simulink model "ACC"  (R2020b)
settings: Solver=VariableStepAuto  StartTime=0.0  StopTime=500  RelTol=1e-3
values from neighbouring files (symbols this model uses):
  plant_den = [1 1/50.531]    [ACC_Script.m]
  plant_num = 9.2251*1e-4    (= 0.00092251)    [ACC_Script.m]    (also in Cruise_Control_design.m; Headway_Controller_Design.m = 0.00092212)
undefined symbols (not defined in the file or in its folder): sigbuilder_block
libraries: pid_lib x2
settings Model: Creator=ChOm1  LastModifiedBy=ChOm1

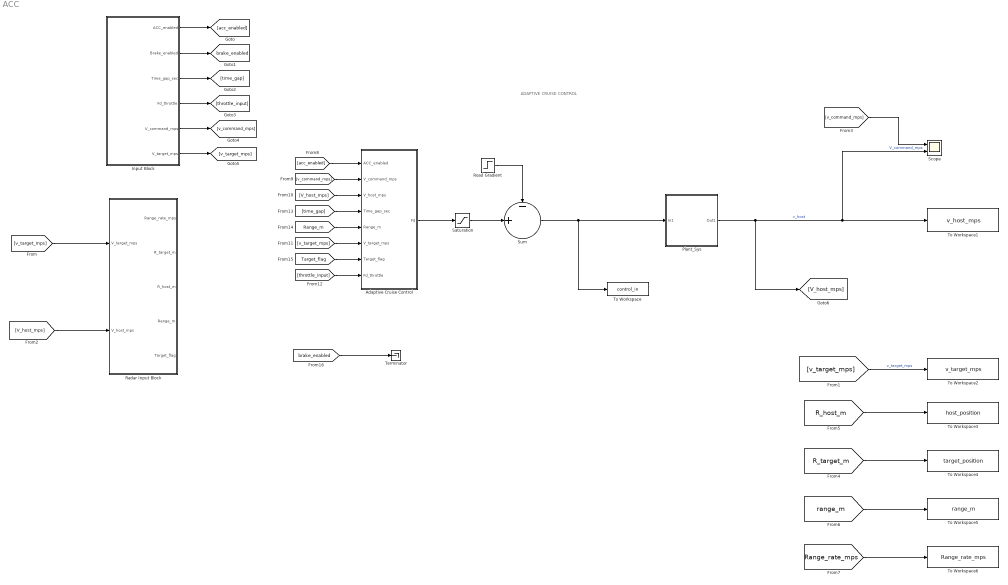
== system ACC ==
  note: ADAPTIVE CRUISE CONTROL
  Adaptive Cruise Control : Subsystem
  Input Block : Subsystem
  Plant_Sys : Subsystem
  Radar Input Block : Subsystem
  Road Gradient : Step  SampleTime=0
  Saturation : Saturate  UpperLimit=1000  LowerLimit=-1000
  Scope : Scope  NumInputPorts=2
  Sum : Sum  Inputs=-+|
  Terminator : Terminator
  To Workspace : ToWorkspace  VariableName=control_in  SaveFormat=Timeseries  SampleTime=-1
  To Workspace1 : ToWorkspace  VariableName=v_host_mps  SaveFormat=Timeseries  SampleTime=-1
  To Workspace2 : ToWorkspace  VariableName=v_target_mps  SaveFormat=Timeseries  SampleTime=-1
  To Workspace3 : ToWorkspace  VariableName=host_position  SaveFormat=Timeseries  SampleTime=-1
  To Workspace4 : ToWorkspace  VariableName=target_position  SaveFormat=Timeseries  SampleTime=-1
  To Workspace5 : ToWorkspace  VariableName=range_m  SaveFormat=Timeseries  SampleTime=-1
  To Workspace6 : ToWorkspace  VariableName=Range_rate_mps  SaveFormat=Timeseries  SampleTime=-1
  tag scope: brake_enabled=global
  wires:
  Input Block/1(ACC_enabled) -> [acc_enabled]
  Input Block/2(Brake_enabled) -> [brake_enabled]
  Input Block/3(Time_gap_sec) -> [time_gap]
  Input Block/4(Fd_throttle) -> [throttle_input]
  Input Block/5(V_command_mps) -> [v_command_mps]
  Input Block/6(V_target_mps) -> [v_target_mps]
  [v_target_mps] -> Radar Input Block/1(V_target_mps)
  Adaptive Cruise Control/1(Fd) -> Saturation/1
  Saturation/1 -> Sum/2
  Road Gradient/1 -> Sum/1
  Plant_Sys/1(Out1) -> [V_host_mps], Scope/2, To Workspace1/1  "v_host"
  [v_target_mps] -> To Workspace2/1  "v_target_mps"
  [v_command_mps] -> Scope/1  "V_command_mps"
  [R_target_m] -> To Workspace4/1
  [R_host_m] -> To Workspace3/1
  [range_m] -> To Workspace5/1
  [Range_rate_mps] -> To Workspace6/1
  [acc_enabled] -> Adaptive Cruise Control/1(ACC_enabled)
  [v_command_mps] -> Adaptive Cruise Control/2(V_command_mps)
  [V_host_mps] -> Adaptive Cruise Control/3(V_host_mps)
  [v_target_mps] -> Adaptive Cruise Control/6(V_target_mps)
  [throttle_input] -> Adaptive Cruise Control/8(Fd_throttle)
  [time_gap] -> Adaptive Cruise Control/4(Time_gap_sec)
  [Range_m] -> Adaptive Cruise Control/5(Range_m)
  [Target_flag] -> Adaptive Cruise Control/7(Target_flag)
  [brake_enabled] -> Terminator/1
  Sum/1 -> Plant_Sys/1(In1), To Workspace/1
  [V_host_mps] -> Radar Input Block/2(V_host_mps)

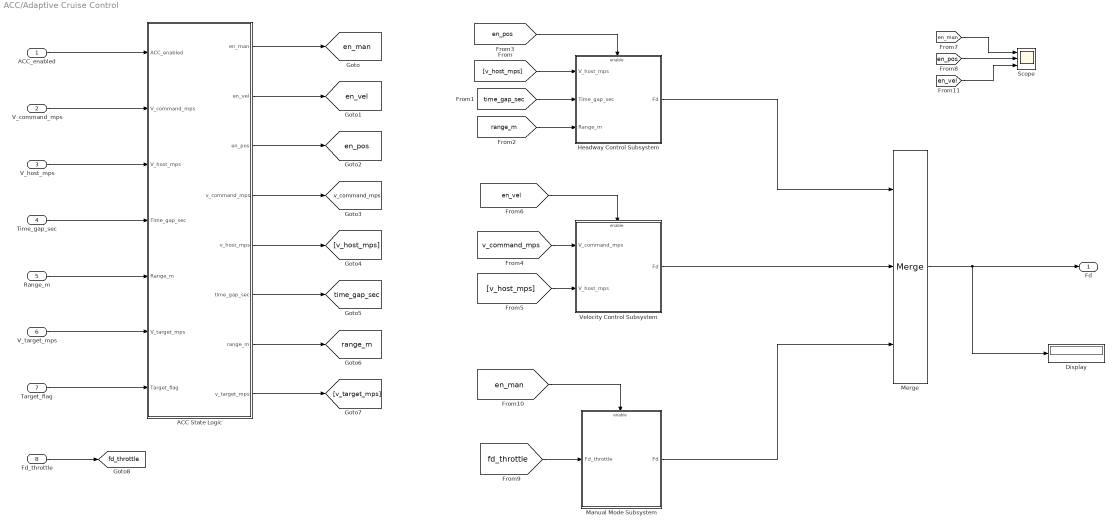
== system ACC/Adaptive Cruise Control ==
  ACC_enabled : Inport
  V_command_mps : Inport  Port=2
  V_host_mps : Inport  Port=3
  Time_gap_sec : Inport  Port=4
  Range_m : Inport  Port=5
  V_target_mps : Inport  Port=6
  Target_flag : Inport  Port=7
  Fd_throttle : Inport  Port=8
  ACC State Logic : Subsystem
  Display : Display
  Headway Control Subsystem : Subsystem
  Manual Mode Subsystem : Subsystem
  Merge : Merge  Inputs=3
  Scope : Scope  NumInputPorts=3
  Velocity Control Subsystem : Subsystem
  Fd : Outport
  tag scope: en_man=global, en_pos=global, en_vel=global, fd_throttle=global, range_m=global, time_gap_sec=global, v_command_mps=global
  wires:
  ACC_enabled/1 -> ACC State Logic/1(ACC_enabled)
  V_command_mps/1 -> ACC State Logic/2(V_command_mps)
  V_host_mps/1 -> ACC State Logic/3(V_host_mps)
  Time_gap_sec/1 -> ACC State Logic/4(Time_gap_sec)
  Range_m/1 -> ACC State Logic/5(Range_m)
  V_target_mps/1 -> ACC State Logic/6(V_target_mps)
  Target_flag/1 -> ACC State Logic/7(Target_flag)
  ACC State Logic/1(en_man) -> [en_man]
  ACC State Logic/2(en_vel) -> [en_vel]
  ACC State Logic/3(en_pos) -> [en_pos]
  ACC State Logic/4(v_command_mps) -> [v_command_mps]
  ACC State Logic/5(v_host_mps) -> [v_host_mps]
  ACC State Logic/6(time_gap_sec) -> [time_gap_sec]
  ACC State Logic/7(range_m) -> [range_m]
  ACC State Logic/8(v_target_mps) -> [v_target_mps]
  [v_host_mps] -> Headway Control Subsystem/1(V_host_mps)
  [time_gap_sec] -> Headway Control Subsystem/2(Time_gap_sec)
  [range_m] -> Headway Control Subsystem/3(Range_m)
  [en_pos] -> Headway Control Subsystem/Enable
  [v_command_mps] -> Velocity Control Subsystem/1(V_command_mps)
  [v_host_mps] -> Velocity Control Subsystem/2(V_host_mps)
  [en_vel] -> Velocity Control Subsystem/Enable
  Fd_throttle/1 -> [fd_throttle]
  [fd_throttle] -> Manual Mode Subsystem/1(Fd_throttle)
  [en_man] -> Manual Mode Subsystem/Enable
  Headway Control Subsystem/1(Fd) -> Merge/1
  Velocity Control Subsystem/1(Fd) -> Merge/2
  Manual Mode Subsystem/1(Fd) -> Merge/3
  Merge/1 -> Display/1, Fd/1
  [en_man] -> Scope/1
  [en_pos] -> Scope/2
  [en_vel] -> Scope/3

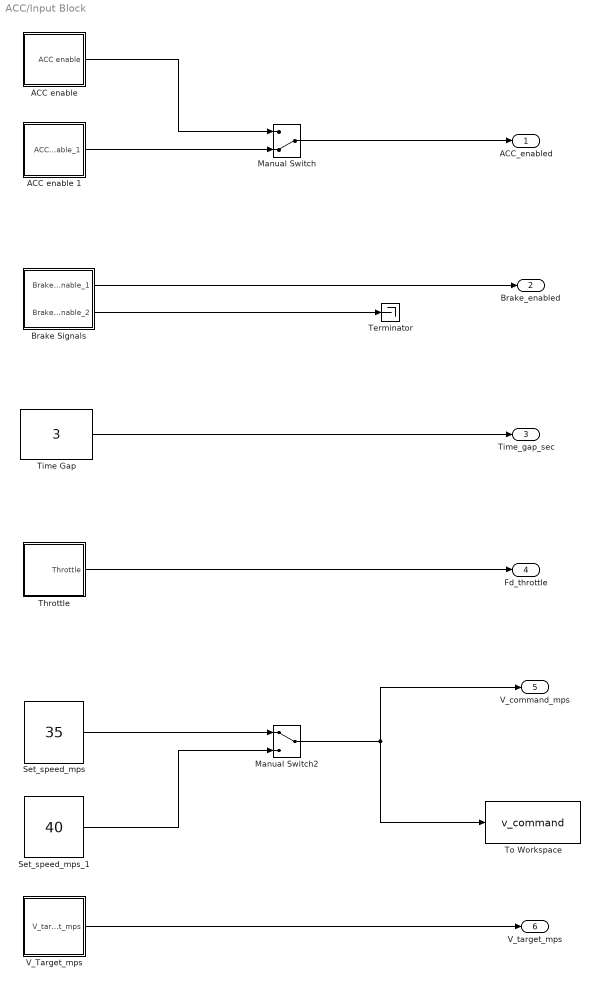
== system ACC/Input Block ==
  ACC enable : Subsystem  Tag=STV Subsys  LoadFcn=sigbuilder_block('load');  StartFcn=sigbuilder_block('start');  StopFcn=sigbuilder_block('stop');  ClipboardFcn=sigbuilder_block('clipboard');  mask(Sigbuilder block){tuvar=[0:10]}
      mask help: Simulink:masks:SigbuilderBlock_MD
      mask init:
      | if ~strcmp(get_param(bdroot(gcbh),'SimulationStatus'),'stopped') tuvar = sigbuilder_block('maskInit'); end
      settings: CopyFcn=sigbuilder_block('copy');  DeleteFcn=sigbuilder_block('delete');  ModelCloseFcn=sigbuilder_block('modelClose');  PreSaveFcn=sigbuilder_block('preSave');  PauseFcn=sigbuilder_block('pause');  ContinueFcn=sigbuilder_block('continue');  NameChangeFcn=sigbuilder_block('namechange');  OpenFcn=sigbuilder_block('open',[172.5 40 550.5 362.5 ]);  CloseFcn=sigbuilder_block('close');
      mask Display: plot(0, 0, 100, 100,[2, 2, 32, 32, 2], [68, 8, 8, 68, 68],[32, 2], [38, 38], [32, 19, 2],[53, 60, 44], [32, 17, 17, 2],[16, 16, 31, 31]);txt = getActiveGroup(gcbh);text(2, 100, txt,'verticalAlignment', 'top');
  ACC enable 1 : Subsystem  Tag=STV Subsys  LoadFcn=sigbuilder_block('load');  StartFcn=sigbuilder_block('start');  StopFcn=sigbuilder_block('stop');  ClipboardFcn=sigbuilder_block('clipboard');  mask(Sigbuilder block){tuvar=[0:10]}
      mask help: Simulink:masks:SigbuilderBlock_MD
      mask init:
      | if ~strcmp(get_param(bdroot(gcbh),'SimulationStatus'),'stopped') tuvar = sigbuilder_block('maskInit'); end
      settings: CopyFcn=sigbuilder_block('copy');  DeleteFcn=sigbuilder_block('delete');  ModelCloseFcn=sigbuilder_block('modelClose');  PreSaveFcn=sigbuilder_block('preSave');  PauseFcn=sigbuilder_block('pause');  ContinueFcn=sigbuilder_block('continue');  NameChangeFcn=sigbuilder_block('namechange');  OpenFcn=sigbuilder_block('open',[427 63 479.5 302.5 ]);  CloseFcn=sigbuilder_block('close');
      mask Display: plot(0, 0, 100, 100,[2, 2, 32, 32, 2], [68, 8, 8, 68, 68],[32, 2], [38, 38], [32, 19, 2],[53, 60, 44], [32, 17, 17, 2],[16, 16, 31, 31]);txt = getActiveGroup(gcbh);text(2, 100, txt,'verticalAlignment', 'top');
  Brake Signals : Subsystem  Tag=STV Subsys  LoadFcn=sigbuilder_block('load');  StartFcn=sigbuilder_block('start');  StopFcn=sigbuilder_block('stop');  ClipboardFcn=sigbuilder_block('clipboard');  mask(Sigbuilder block){tuvar=[0:10]}
      mask help: Simulink:masks:SigbuilderBlock_MD
      mask init:
      | if ~strcmp(get_param(bdroot(gcbh),'SimulationStatus'),'stopped') tuvar = sigbuilder_block('maskInit'); end
      settings: CopyFcn=sigbuilder_block('copy');  DeleteFcn=sigbuilder_block('delete');  ModelCloseFcn=sigbuilder_block('modelClose');  PreSaveFcn=sigbuilder_block('preSave');  PauseFcn=sigbuilder_block('pause');  ContinueFcn=sigbuilder_block('continue');  NameChangeFcn=sigbuilder_block('namechange');  OpenFcn=sigbuilder_block('open',[87.5 9 430.5 307 ]);  CloseFcn=sigbuilder_block('close');
      mask Display: plot(0, 0, 100, 100,[2, 2, 32, 32, 2], [68, 8, 8, 68, 68],[32, 2], [38, 38], [32, 19, 2],[53, 60, 44], [32, 17, 17, 2],[16, 16, 31, 31]);txt = getActiveGroup(gcbh);text(2, 100, txt,'verticalAlignment', 'top');
  Manual Switch : ManualSwitch  CurrentSetting=0
  Manual Switch2 : ManualSwitch
  Set_speed_mps : Constant  Value=35
  Set_speed_mps_1 : Constant  Value=40
  Terminator : Terminator
  Throttle : Subsystem  Tag=STV Subsys  LoadFcn=sigbuilder_block('load');  StartFcn=sigbuilder_block('start');  StopFcn=sigbuilder_block('stop');  ClipboardFcn=sigbuilder_block('clipboard');  mask(Sigbuilder block){tuvar=[0:10]}
      mask help: Simulink:masks:SigbuilderBlock_MD
      mask init:
      | if ~strcmp(get_param(bdroot(gcbh),'SimulationStatus'),'stopped') tuvar = sigbuilder_block('maskInit'); end
      settings: CopyFcn=sigbuilder_block('copy');  DeleteFcn=sigbuilder_block('delete');  ModelCloseFcn=sigbuilder_block('modelClose');  PreSaveFcn=sigbuilder_block('preSave');  PauseFcn=sigbuilder_block('pause');  ContinueFcn=sigbuilder_block('continue');  NameChangeFcn=sigbuilder_block('namechange');  OpenFcn=sigbuilder_block('open',[172.5 40 550.5 362.5 ]);  CloseFcn=sigbuilder_block('close');
      mask Display: plot(0, 0, 100, 100,[2, 2, 32, 32, 2], [68, 8, 8, 68, 68],[32, 2], [38, 38], [32, 19, 2],[53, 60, 44], [32, 17, 17, 2],[16, 16, 31, 31]);txt = getActiveGroup(gcbh);text(2, 100, txt,'verticalAlignment', 'top');
  Time Gap : Constant  Value=3
  To Workspace : ToWorkspace  VariableName=v_command  SaveFormat=Timeseries  SampleTime=-1
  V_Target_mps : Subsystem  Tag=STV Subsys  LoadFcn=sigbuilder_block('load');  StartFcn=sigbuilder_block('start');  StopFcn=sigbuilder_block('stop');  ClipboardFcn=sigbuilder_block('clipboard');  mask(Sigbuilder block){tuvar=[0:10]}
      mask help: Simulink:masks:SigbuilderBlock_MD
      mask init:
      | if ~strcmp(get_param(bdroot(gcbh),'SimulationStatus'),'stopped') tuvar = sigbuilder_block('maskInit'); end
      settings: CopyFcn=sigbuilder_block('copy');  DeleteFcn=sigbuilder_block('delete');  ModelCloseFcn=sigbuilder_block('modelClose');  PreSaveFcn=sigbuilder_block('preSave');  PauseFcn=sigbuilder_block('pause');  ContinueFcn=sigbuilder_block('continue');  NameChangeFcn=sigbuilder_block('namechange');  OpenFcn=sigbuilder_block('open',[5.5 30 949 418 ]);  CloseFcn=sigbuilder_block('close');
      mask Display: plot(0, 0, 100, 100,[2, 2, 32, 32, 2], [68, 8, 8, 68, 68],[32, 2], [38, 38], [32, 19, 2],[53, 60, 44], [32, 17, 17, 2],[16, 16, 31, 31]);txt = getActiveGroup(gcbh);text(2, 100, txt,'verticalAlignment', 'top');
  ACC_enabled : Outport
  Brake_enabled : Outport  Port=2
  Time_gap_sec : Outport  Port=3
  Fd_throttle : Outport  Port=4
  V_command_mps : Outport  Port=5
  V_target_mps : Outport  Port=6
  wires:
  Manual Switch/1 -> ACC_enabled/1
  Brake Signals/1(Brake_enable_1) -> Brake_enabled/1
  Brake Signals/2(Brake_enable_2) -> Terminator/1
  Time Gap/1 -> Time_gap_sec/1
  Throttle/1(Throttle) -> Fd_throttle/1
  V_Target_mps/1(V_target_mps) -> V_target_mps/1
  ACC enable/1(ACC enable) -> Manual Switch/1
  ACC enable 1/1(ACC_enable_1) -> Manual Switch/2
  Set_speed_mps/1 -> Manual Switch2/1
  Manual Switch2/1 -> To Workspace/1, V_command_mps/1
  Set_speed_mps_1/1 -> Manual Switch2/2

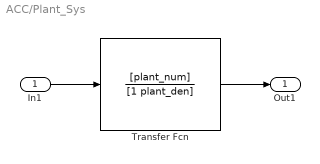
== system ACC/Plant_Sys ==
  In1 : Inport
  Transfer Fcn : TransferFcn  Numerator=[plant_num]  Denominator=[1 plant_den]
  Out1 : Outport
  wires:
  In1/1 -> Transfer Fcn/1
  Transfer Fcn/1 -> Out1/1

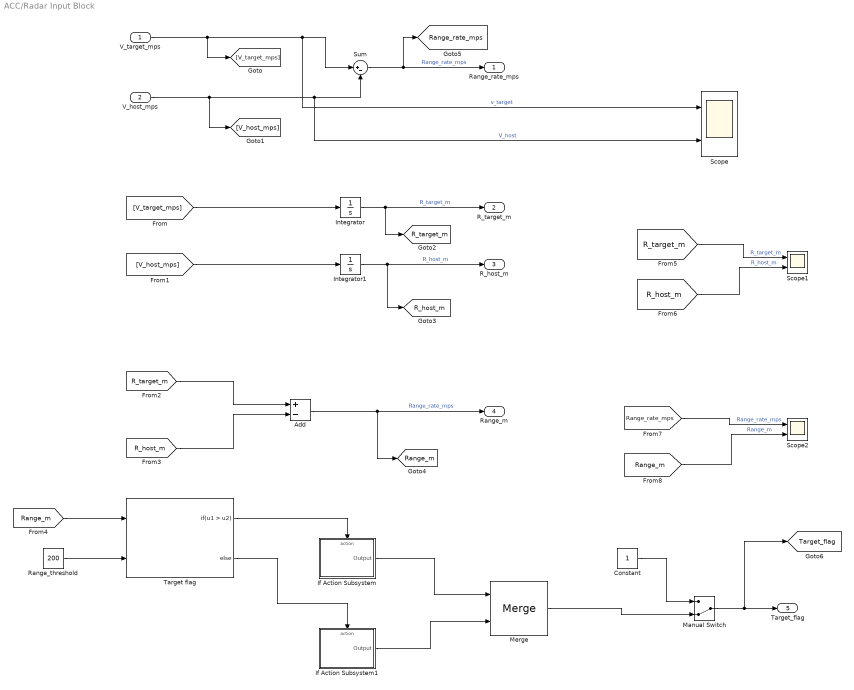
== system ACC/Radar Input Block ==
  V_target_mps : Inport
  V_host_mps : Inport  Port=2
  Add : Sum  Inputs=+-
  Constant : Constant
  If Action Subsystem : Subsystem  TreatAsAtomicUnit=on
  If Action Subsystem1 : Subsystem  TreatAsAtomicUnit=on
  Integrator : Integrator  InitialCondition=500
  Integrator1 : Integrator
  Manual Switch : ManualSwitch  CurrentSetting=0
  Merge : Merge
  Range_threshold : Constant  Value=200
  Scope : Scope  NumInputPorts=2
  Scope1 : Scope  NumInputPorts=2
  Scope2 : Scope  NumInputPorts=2
  Sum : Sum  Inputs=|+-
  "Target flag " : If  NumInputs=2  IfExpression=u1 > u2
  Range_rate_mps : Outport
  R_target_m : Outport  Port=2
  R_host_m : Outport  Port=3
  Range_m : Outport  Port=4
  Target_flag : Outport  Port=5
  tag scope: R_host_m=global, R_target_m=global, Range_m=global, Range_rate_mps=global, Target_flag=global
  wires:
  V_host_mps/1 -> [V_host_mps], Scope/2, Sum/2  "V_host"
  V_target_mps/1 -> Scope/1, Sum/1, [V_target_mps]  "v_target"
  Sum/1 -> [Range_rate_mps], Range_rate_mps/1  "Range_rate_mps"
  [V_target_mps] -> Integrator/1
  [V_host_mps] -> Integrator1/1
  Integrator1/1 -> [R_host_m], R_host_m/1  "R_host_m"
  Integrator/1 -> [R_target_m], R_target_m/1  "R_target_m"
  [R_target_m] -> Add/1
  [R_host_m] -> Add/2
  Add/1 -> [Range_m], Range_m/1  "Range_rate_mps"
  Range_threshold/1 -> "Target flag "/2
  [Range_m] -> "Target flag "/1
  "Target flag "/1 -> If Action Subsystem/Action
  "Target flag "/2 -> If Action Subsystem1/Action
  If Action Subsystem/1(Output) -> Merge/1
  If Action Subsystem1/1(Output) -> Merge/2
  Manual Switch/1 -> [Target_flag], Target_flag/1
  Constant/1 -> Manual Switch/1
  Merge/1 -> Manual Switch/2
  [R_target_m] -> Scope1/1  "R_target_m"
  [R_host_m] -> Scope1/2  "R_host_m"
  [Range_rate_mps] -> Scope2/1  "Range_rate_mps"
  [Range_m] -> Scope2/2  "Range_m"

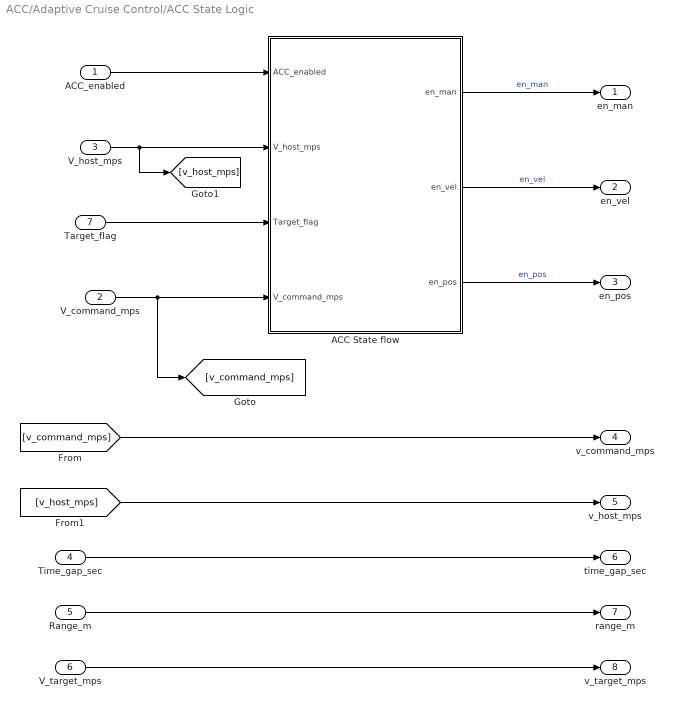
== system ACC/Adaptive Cruise Control/ACC State Logic ==
  ACC_enabled : Inport
  V_command_mps : Inport  Port=2
  V_host_mps : Inport  Port=3
  Time_gap_sec : Inport  Port=4
  Range_m : Inport  Port=5
  V_target_mps : Inport  Port=6
  Target_flag : Inport  Port=7
  ACC State flow : Stateflow chart  TreatAsAtomicUnit=on
  en_man : Outport
  en_vel : Outport  Port=2
  en_pos : Outport  Port=3
  v_command_mps : Outport  Port=4
  v_host_mps : Outport  Port=5
  time_gap_sec : Outport  Port=6
  range_m : Outport  Port=7
  v_target_mps : Outport  Port=8
  wires:
  ACC State flow/2(en_vel) -> en_vel/1  "en_vel"
  ACC State flow/3(en_pos) -> en_pos/1  "en_pos"
  [v_command_mps] -> v_command_mps/1
  [v_host_mps] -> v_host_mps/1
  Time_gap_sec/1 -> time_gap_sec/1
  Range_m/1 -> range_m/1
  V_target_mps/1 -> v_target_mps/1
  ACC State flow/1(en_man) -> en_man/1  "en_man"
  ACC_enabled/1 -> ACC State flow/1(ACC_enabled)
  Target_flag/1 -> ACC State flow/3(Target_flag)
  V_host_mps/1 -> [v_host_mps], ACC State flow/2(V_host_mps)
  V_command_mps/1 -> [v_command_mps], ACC State flow/4(V_command_mps)

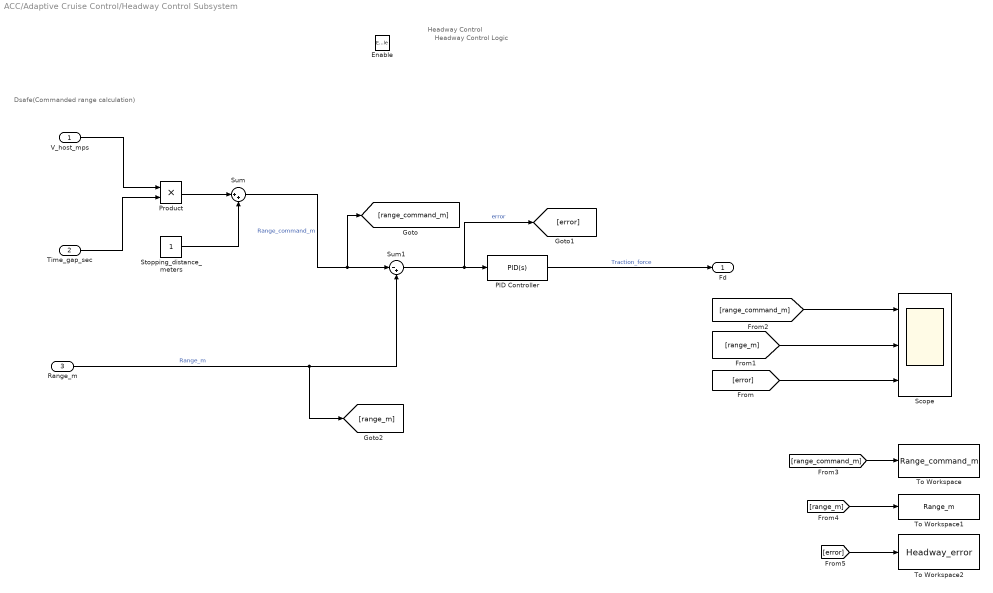
== system ACC/Adaptive Cruise Control/Headway Control Subsystem ==
  note: Headway Control Logic
  note: Headway Control
  note: Dsafe(Commanded range calculation)
  V_host_mps : Inport
  Time_gap_sec : Inport  Port=2
  Range_m : Inport  Port=3
  Enable : EnablePort
  PID Controller : pid_lib/PID Controller  Controller=PID  Form=Parallel  TimeDomain=Continuous-time  UseExternalTs=off  SampleTime=-1  IntegratorMethod=Forward Euler  FilterMethod=Forward Euler  ControllerParametersSource=internal  P=1.23373996546318  I=0.00611903694432425  D=34.7378082281947  UseFilter=on  N=75  TunerSelectOption=Transfer Function Based (PID Tuner App)  InitialConditionSource=internal  InitialConditionForIntegrator=0  InitialConditionForFilter=0  DifferentiatorICPrevScaledInput=0  ExternalReset=none  TrackingMode=off  Kt=1  LimitOutput=off  SatLimitsSource=internal  UpperSaturationLimit=inf  LowerSaturationLimit=-inf  LinearizeAsGain=on  AntiWindupMode=none  Kb=1  POutMin=[]  POutMax=[]  IOutMin=[]  IOutMax=[]  DOutMin=[]  DOutMax=[]  NOutMin=[]  NOutMax=[]  SumOutMin=[]  SumOutMax=[]  SaturationOutMin=[]  SaturationOutMax=[]  PParamMin=[]  PParamMax=[]  IParamMin=[]  IParamMax=[]  DParamMin=[]  DParamMax=[]  NParamMin=[]  NParamMax=[]  KbParamMin=[]  KbParamMax=[]  KtParamMin=[]  KtParamMax=[]  KbOutMin=[]  KbOutMax=[]  KtOutMin=[]  KtOutMax=[]  IntegratorOutMin=[]  IntegratorOutMax=[]  FilterOutMin=[]  FilterOutMax=[]  SumI1OutMin=[]  SumI1OutMax=[]  SumI2OutMin=[]  SumI2OutMax=[]  SumI3OutMin=[]  SumI3OutMax=[]  SumI4OutMin=[]  SumI4OutMax=[]  SumDOutMin=[]  SumDOutMax=[]  DifferentiatorOutMin=[]  DifferentiatorOutMax=[]  FilterDiffOutCoefMin=[]  FilterDiffOutCoefMax=[]  ReciprocalOutMin=[]  ReciprocalOutMax=[]  SumDenOutMin=[]  SumDenOutMax=[]  SumNumOutMin=[]  SumNumOutMax=[]  DivideOutMin=[]  DivideOutMax=[]  UdiffTsProdOutMin=[]  UdiffTsProdOutMax=[]  NTsProdOutMin=[]  NTsProdOutMax=[]  UintegralTsProdOutMin=[]  UintegralTsProdOutMax=[]  UngainTsProdOutMin=[]  UngainTsProdOutMax=[]  IntegratorContinuousStateAttributes=''  IntegratorStateMustResolveToSignalObject=off  IntegratorRTWStateStorageClass=Auto  FilterContinuousStateAttributes=''  FilterStateMustResolveToSignalObject=off  FilterRTWStateStorageClass=Auto  ParallelPVariant=InternalParameters  IdealPVariant=Disabled  IVariant=InternalParameters  DVariant=InternalParameters  IntegratorVariant=Continuous  SatVariant=Disabled  AWVariant=Passthrough  PCopyVariant=Disabled  TRVariant=Disabled  FdbkBlocksVariant=Forward  IdealPFdbkVariant=Disabled  SatFdbkVariant=Disabled  DerivativeFilterVariant=ContFilter  NVariant=InternalParameters  NCopyVariant=Disabled  FilterICVariant=InternalICsFilter  IntegratorICVariant=InternalICs  ExternalResetVariant=Disabled  TRSumVariant=Passthrough  SumFdbkVariant=Disabled  SumVariant=Sum_PID  TsampFilterVariant=InternalTs  TsampNgainVariant=Passthrough  TsampIntegralVariant=Passthrough  ExternalSaturationOutDataTypeStr=Inherit: Same as second input
  Product : Product
  Scope : Scope  NumInputPorts=3
  Stopping_distance_meters : Constant
  Sum : Sum  Inputs=|++
  Sum1 : Sum  Inputs=|-+
  To Workspace : ToWorkspace  VariableName=Range_command_m  SampleTime=-1
  To Workspace1 : ToWorkspace  VariableName=Range_m  SampleTime=-1
  To Workspace2 : ToWorkspace  VariableName=Headway_error  SaveFormat=Timeseries  SampleTime=-1
  Fd : Outport
  wires:
  [range_m] -> To Workspace1/1
  [error] -> Scope/3
  [error] -> To Workspace2/1
  [range_command_m] -> Scope/1
  [range_m] -> Scope/2
  [range_command_m] -> To Workspace/1
  PID Controller/1 -> Fd/1  "Traction_force"
  Sum/1 -> [range_command_m], Sum1/1  "Range_command_m"
  Stopping_distance_meters/1 -> Sum/2
  V_host_mps/1 -> Product/1
  Sum1/1 -> [error], PID Controller/1  "error"
  Time_gap_sec/1 -> Product/2
  Range_m/1 -> [range_m], Sum1/2  "Range_m"
  Product/1 -> Sum/1

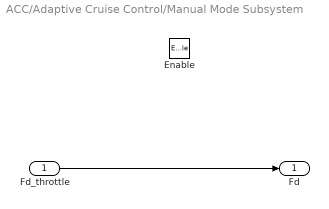
== system ACC/Adaptive Cruise Control/Manual Mode Subsystem ==
  Fd_throttle : Inport
  Enable : EnablePort
  Fd : Outport
  wires:
  Fd_throttle/1 -> Fd/1

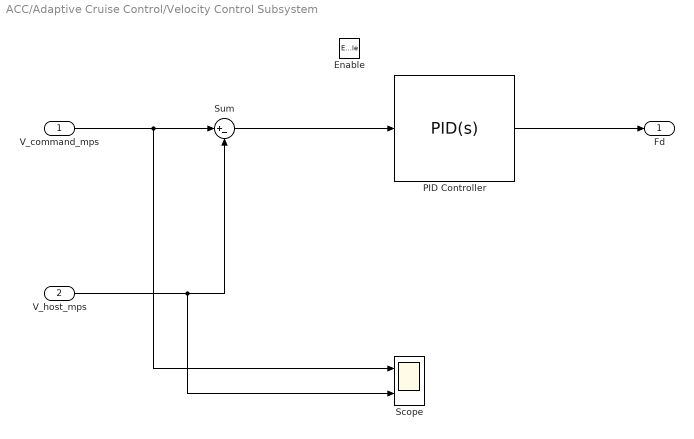
== system ACC/Adaptive Cruise Control/Velocity Control Subsystem ==
  V_command_mps : Inport
  V_host_mps : Inport  Port=2
  Enable : EnablePort
  PID Controller : pid_lib/PID Controller  Controller=PID  Form=Parallel  TimeDomain=Continuous-time  UseExternalTs=off  SampleTime=-1  IntegratorMethod=Forward Euler  FilterMethod=Forward Euler  ControllerParametersSource=internal  P=174.6119  I=10.1187  D=247.7833  UseFilter=on  N=100  TunerSelectOption=Transfer Function Based (PID Tuner App)  InitialConditionSource=internal  InitialConditionForIntegrator=0  InitialConditionForFilter=0  DifferentiatorICPrevScaledInput=0  ExternalReset=none  TrackingMode=off  Kt=1  LimitOutput=off  SatLimitsSource=internal  UpperSaturationLimit=inf  LowerSaturationLimit=-inf  LinearizeAsGain=on  AntiWindupMode=none  Kb=1  POutMin=[]  POutMax=[]  IOutMin=[]  IOutMax=[]  DOutMin=[]  DOutMax=[]  NOutMin=[]  NOutMax=[]  SumOutMin=[]  SumOutMax=[]  SaturationOutMin=[]  SaturationOutMax=[]  PParamMin=[]  PParamMax=[]  IParamMin=[]  IParamMax=[]  DParamMin=[]  DParamMax=[]  NParamMin=[]  NParamMax=[]  KbParamMin=[]  KbParamMax=[]  KtParamMin=[]  KtParamMax=[]  KbOutMin=[]  KbOutMax=[]  KtOutMin=[]  KtOutMax=[]  IntegratorOutMin=[]  IntegratorOutMax=[]  FilterOutMin=[]  FilterOutMax=[]  SumI1OutMin=[]  SumI1OutMax=[]  SumI2OutMin=[]  SumI2OutMax=[]  SumI3OutMin=[]  SumI3OutMax=[]  SumI4OutMin=[]  SumI4OutMax=[]  SumDOutMin=[]  SumDOutMax=[]  DifferentiatorOutMin=[]  DifferentiatorOutMax=[]  FilterDiffOutCoefMin=[]  FilterDiffOutCoefMax=[]  ReciprocalOutMin=[]  ReciprocalOutMax=[]  SumDenOutMin=[]  SumDenOutMax=[]  SumNumOutMin=[]  SumNumOutMax=[]  DivideOutMin=[]  DivideOutMax=[]  UdiffTsProdOutMin=[]  UdiffTsProdOutMax=[]  NTsProdOutMin=[]  NTsProdOutMax=[]  UintegralTsProdOutMin=[]  UintegralTsProdOutMax=[]  UngainTsProdOutMin=[]  UngainTsProdOutMax=[]  IntegratorContinuousStateAttributes=''  IntegratorStateMustResolveToSignalObject=off  IntegratorRTWStateStorageClass=Auto  FilterContinuousStateAttributes=''  FilterStateMustResolveToSignalObject=off  FilterRTWStateStorageClass=Auto  ParallelPVariant=InternalParameters  IdealPVariant=Disabled  IVariant=InternalParameters  DVariant=InternalParameters  IntegratorVariant=Continuous  SatVariant=Disabled  AWVariant=Passthrough  PCopyVariant=Disabled  TRVariant=Disabled  FdbkBlocksVariant=Forward  IdealPFdbkVariant=Disabled  SatFdbkVariant=Disabled  DerivativeFilterVariant=ContFilter  NVariant=InternalParameters  NCopyVariant=Disabled  FilterICVariant=InternalICsFilter  IntegratorICVariant=InternalICs  ExternalResetVariant=Disabled  TRSumVariant=Passthrough  SumFdbkVariant=Disabled  SumVariant=Sum_PID  TsampFilterVariant=InternalTs  TsampNgainVariant=Passthrough  TsampIntegralVariant=Passthrough  ExternalSaturationOutDataTypeStr=Inherit: Same as second input
  Scope : Scope  NumInputPorts=2
  Sum : Sum  Inputs=|+-
  Fd : Outport
  wires:
  V_host_mps/1 -> Scope/2, Sum/2
  V_command_mps/1 -> Scope/1, Sum/1
  Sum/1 -> PID Controller/1
  PID Controller/1 -> Fd/1

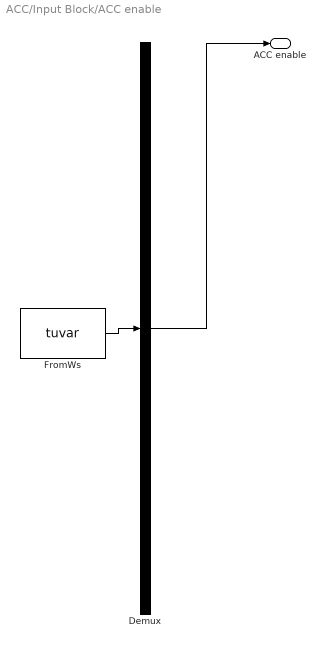
== system ACC/Input Block/ACC enable ==
  Demux : Demux  Tag=STV Demux  Outputs=1
      settings: DisplayOption=none
  FromWs : FromWorkspace  Tag=STV FromWs  VariableName=tuvar
      SigBuilderData=|
      | common.afterFinalStr = 'Extrapolate'
      | common.sampleTime = 0
      | dataSet.timeRange = [0 500]
      | dataSet.name = 'Group 1'
      | sbobj.Groups.Name = 'Group 1'
      | sbobj.Groups.Signals.Name = 'ACC enable'
      | sbobj.Groups.Signals.XData = [0 500]
      | sbobj.Groups.Signals.YData = [0.99 0.99]
      | sbobj.Groups.TimeRange = [0 500]
  ACC enable : Outport  Tag=STV Outport
  wires:
  FromWs/1 -> Demux/1
  Demux/1 -> ACC enable/1

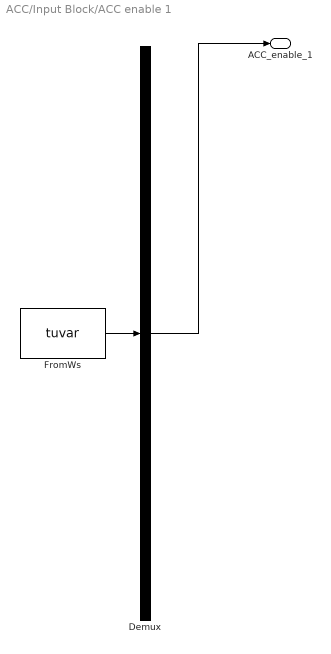
== system ACC/Input Block/ACC enable 1 ==
  Demux : Demux  Tag=STV Demux  Outputs=1
      settings: DisplayOption=none
  FromWs : FromWorkspace  Tag=STV FromWs  VariableName=tuvar
      SigBuilderData=|
      | common.afterFinalStr = 'Extrapolate'
      | common.sampleTime = 0
      | dataSet.timeRange = [0 500]
      | dataSet.name = 'Group 1'
      | sbobj.Groups.Name = 'Group 1'
      | sbobj.Groups.Signals.Name = 'ACC_enable_1'
      | sbobj.Groups.Signals.XData = [0 4 4 350 350 500]
      | sbobj.Groups.Signals.YData = [0 0 1 1 0 0]
      | sbobj.Groups.TimeRange = [0 500]
  ACC_enable_1 : Outport  Tag=STV Outport
  wires:
  Demux/1 -> ACC_enable_1/1
  FromWs/1 -> Demux/1

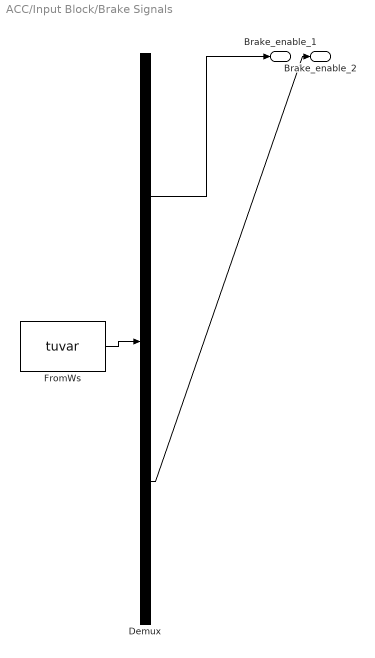
== system ACC/Input Block/Brake Signals ==
  Demux : Demux  Tag=STV Demux  Outputs=2
      settings: DisplayOption=none
  FromWs : FromWorkspace  Tag=STV FromWs  VariableName=tuvar
      SigBuilderData=|
      | common.afterFinalStr = 'Extrapolate'
      | common.sampleTime = 0
      | dataSet.timeRange = [0 500]
      | dataSet.name = 'Group 1'
      | sbobj.Groups.Name = 'Group 1'
      | sbobj.Groups.Signals(1).Name = 'Brake_enable_1'
      | sbobj.Groups.Signals(1).XData = [0 4 255.5 255.5 350 500]
      | sbobj.Groups.Signals(1).YData = [0 0 0 1 1 1]
      | sbobj.Groups.Signals(2).Name = 'Brake_enable_2'
      | sbobj.Groups.Signals(2).XData = [0 500]
      | sbobj.Groups.Signals(2).YData = [0 0]
      | sbobj.Groups.TimeRange = [0 500]
  Brake_enable_1 : Outport  Tag=STV Outport
  Brake_enable_2 : Outport  Tag=STV Outport  Port=2
  wires:
  Demux/1 -> Brake_enable_1/1
  FromWs/1 -> Demux/1
  Demux/2 -> Brake_enable_2/1

== system ACC/Input Block/Throttle ==
  Demux : Demux  Tag=STV Demux  Outputs=1
      settings: DisplayOption=none
  FromWs : FromWorkspace  Tag=STV FromWs  VariableName=tuvar
      SigBuilderData=|
      | common.afterFinalStr = 'Extrapolate'
      | common.sampleTime = 0
      | dataSet.timeRange = [0 500]
      | dataSet.name = 'Group 1'
      | sbobj.Groups.Name = 'Group 1'
      | sbobj.Groups.Signals.Name = 'Throttle'
      | sbobj.Groups.Signals.XData = [0 500]
      | sbobj.Groups.Signals.YData = [0.99 0.99]
      | sbobj.Groups.TimeRange = [0 500]
  Throttle : Outport  Tag=STV Outport
  wires:
  Demux/1 -> Throttle/1
  FromWs/1 -> Demux/1

== system ACC/Input Block/V_Target_mps ==
  Demux : Demux  Tag=STV Demux  Outputs=1
      settings: DisplayOption=none
  FromWs : FromWorkspace  Tag=STV FromWs  VariableName=tuvar
      SigBuilderData=|
      | common.afterFinalStr = 'Extrapolate'
      | common.sampleTime = 0
      | dataSet.timeRange = [0 500]
      | dataSet.name = 'Group 1'
      | sbobj.Groups.Name = 'Group 1'
      | sbobj.Groups.Signals.Name = 'V_target_mps'
      | sbobj.Groups.Signals.XData = [0 249.5 249.5 300 450 450 500]
      | sbobj.Groups.Signals.YData = [35 35 30 30 30 42 42]
      | sbobj.Groups.TimeRange = [0 500]
  V_target_mps : Outport  Tag=STV Outport
  wires:
  FromWs/1 -> Demux/1
  Demux/1 -> V_target_mps/1

== system ACC/Radar Input Block/If Action Subsystem ==
  Action Port : ActionPort  ActionPortLabel=if(u1 > u2)
  Constant : Constant  Value=0
  Output : Outport
  wires:
  Constant/1 -> Output/1

== system ACC/Radar Input Block/If Action Subsystem1 ==
  Action Port : ActionPort  ActionPortLabel=else
  Constant : Constant
  Output : Outport
  wires:
  Constant/1 -> Output/1

== stateflow chart ACC/Adaptive Cruise Control/ACC State Logic/ACC State flow ==
  state Headway_control
    entry:en_man =false;
    en_vel = false;
    en_pos = true;
  state Velocity_control
    entry:en_man =false;
    en_vel = true;
    en_pos = false;
  state Manual_mode
    entry:en_man =true;
    en_vel = false;
    en_pos = false;
  Manual_mode -> Velocity_control [order 1] : [(ACC_enabled == 1) &&(Target_flag == 0)]
  Headway_control -> Velocity_control [order 2] : [(ACC_enabled == 1) & (Target_flag == 0) || V_host_mps > V_command_mps + 0.5 && after(30,sec)]
  Manual_mode -> Headway_control [order 2] : [(ACC_enabled == 1) && (Target_flag == 1)]
  (default) -> Manual_mode
  Velocity_control -> Manual_mode [order 1] : [(ACC_enabled == 0)]
  Headway_control -> Manual_mode [order 1] : [(ACC_enabled == 0)]
  Velocity_control -> Headway_control [order 2] : [(ACC_enabled == 1) & (Target_flag == 1) && after(30,sec)]
  data: ACC_enabled input; V_host_mps input; Target_flag input; en_man output; en_vel output; en_pos output; V_command_mps input
